simulink subsystem "OnlineID"  (R2021a)
settings: Solver=VariableStepAuto  StartTime=0.0  StopTime=10.0  RelTol=1e-3
(part 1 of 2)
settings Model: Creator=valen  LastModifiedBy=valen

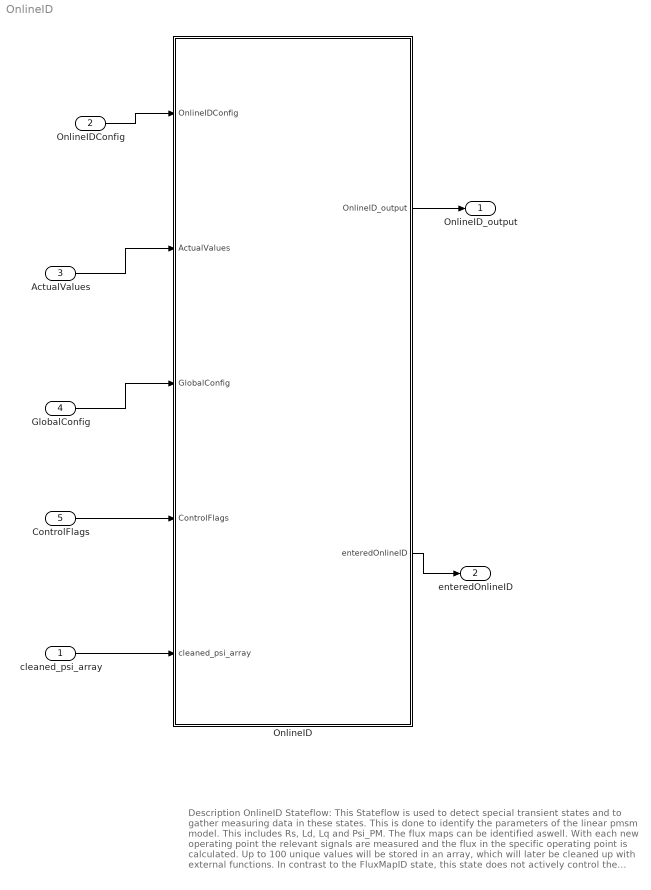
== system OnlineID ==
  note: Description OnlineID Stateflow:
      |
      | This Stateflow is used to detect special transient states and to gather measuring data in these states.
      | This is done to identify the parameters of the linear pmsm model. This includes Rs, Ld, Lq and Psi_PM. The flux maps can be identified aswell. With each new operating point the relevant signals are measured and the flux in the specific operating point is calculated. Up to 100 unique values will be stored in an array, which will later be cleaned up with external functions. In contrast to the FluxMapID state, this state does not actively control the machine via reference currents(except the addition of a injection signal with low amplitude/frequency on top of the reference d-axis current), but therefore measures and calculates the flux in the operating points. This state can therefore run in parallel with your controller, since it does not require full control of the system.
  cleaned_psi_array : Inport
  OnlineIDConfig : Inport  Port=2
  ActualValues : Inport  Port=3
  GlobalConfig : Inport  Port=4
  ControlFlags : Inport  Port=5
  OnlineID : Stateflow chart  TreatAsAtomicUnit=on
      settings: PortSchema="{\"entries\":[{\"content\":{\"sides\":[{\"content\":{\"connectorIds\":[\"In2\",\"In3\",\"In4\",\"In5\",\"In1\"]},\"type\":\"ConnectorPlacement.EquallySpacedRectSide\",\"uuid\":\"7820c6f2-c977-4194-b662-7782d124a170\"},{\"content\":{\"connectorIds\":[\"Out1\",\"Out2\"],\"side\":\"RIGHT\"},\"type\":\"ConnectorPlacement.EquallySpacedRectSide\",\"uuid\":\"8a942b25-9a71-4f6d-9e71-d8e23af023a4\"},{\"content\":{\"connectorIds\":[],\"side\":\"TOP\"},\"type\":\"ConnectorPlacement.EquallySpacedRectSide\",\"uuid\":\"547238ca-03bf-4702-a4be-178f97463404\"}]},\"type\":\"ConnectorPlacement.EquallySpacedConnector\",\"uuid\":\"69f1930a-cf81-42da-9647-066ad6599903\"}],\"packageUris\":[\"http://schema.mathworks.com/mf0/Connector/R2020b\"],\"version\":\"1.0\"}"
  OnlineID_output : Outport
  enteredOnlineID : Outport  Port=2
  wires:
  ControlFlags/1 -> OnlineID/5(ControlFlags)
  GlobalConfig/1 -> OnlineID/4(GlobalConfig)
  OnlineIDConfig/1 -> OnlineID/2(OnlineIDConfig)
  OnlineID/2(enteredOnlineID) -> enteredOnlineID/1
  ActualValues/1 -> OnlineID/3(ActualValues)
  OnlineID/1(OnlineID_output) -> OnlineID_output/1
  cleaned_psi_array/1 -> OnlineID/1(cleaned_psi_array)
